simulink model "ProgrammingCalculator"  (R2021a)
settings: Solver=FixedStepDiscrete  StartTime=0.0  StopTime=10.0  RelTol=1e-3  EnableMultiTasking=on
libraries: simulink x6
settings Model: Creator=Karim  LastModifiedBy=Karim
settings DataIOCC: ReturnWorkspaceOutputs=off
settings OptimizationCC: DefaultParameterBehavior=Inlined  InlineInvariantSignals=on  EnableMemcpy=off  LifeSpan=1  EfficientTunableParamExpr=on
settings DebuggingCC: UnderspecifiedInitializationDetection=Classic  MergeDetectMultiDrivingBlocksExec=none  SFMachineParentedDataDiag=warning  ArithmeticOperatorsInVariantConditions=warning
settings ModelReferenceCC: PropagateSignalLabelsOutOfModel=off
settings SFSimCC: MATLABDynamicMemAlloc=off  CustomCodeUndefinedFunction=UseInterfaceOnly
settings RTWCC: SystemTargetFile=ert.tlc  GenCodeOnly=on  TemplateMakefile=ert_default_tmf  GenerateReport=on  IncludeHyperlinkInReport=on  LaunchReport=on  GenerateTraceInfo=on  GenerateTraceReport=on  GenerateTraceReportSl=on  GenerateTraceReportSf=on  GenerateTraceReportEml=on
settings CodeAppCC: ForceParamTrailComments=on  IgnoreCustomStorageClasses=off  OperatorAnnotations=on  SimulinkDataObjDesc=on  SFDataObjDesc=on  MATLABFcnDesc=on  InsertBlockDesc=on  StateflowObjectComments=on  MATLABSourceComments=on
settings ERTTargetCC: MultiwordLength=2048  GenerateSampleERTMain=on  InlinedParameterPlacement=NonHierarchical  ERTCustomFileTemplate=example_file_process.tlc

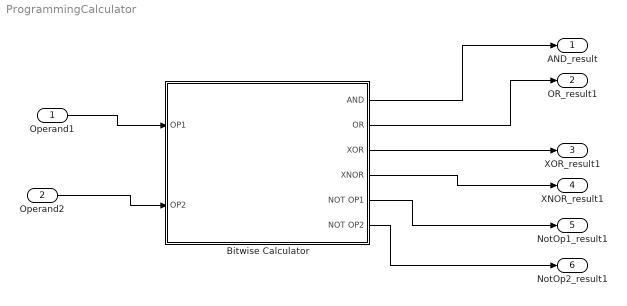
== system ProgrammingCalculator ==
  Operand1 : Inport
  Operand2 : Inport  Port=2
  Bitwise Calculator : Subsystem
  AND_result : Outport
  OR_result1 : Outport  Port=2
  XOR_result1 : Outport  Port=3
  XNOR_result1 : Outport  Port=4
  NotOp1_result1 : Outport  Port=5
  NotOp2_result1 : Outport  Port=6
  wires:
  Bitwise Calculator/1(AND) -> AND_result/1
  Bitwise Calculator/2(OR) -> OR_result1/1
  Bitwise Calculator/3(XOR) -> XOR_result1/1
  Bitwise Calculator/4(XNOR) -> XNOR_result1/1
  Bitwise Calculator/5(NOT OP1) -> NotOp1_result1/1
  Bitwise Calculator/6(NOT OP2) -> NotOp2_result1/1
  Operand1/1 -> Bitwise Calculator/1(OP1)
  Operand2/1 -> Bitwise Calculator/2(OP2)

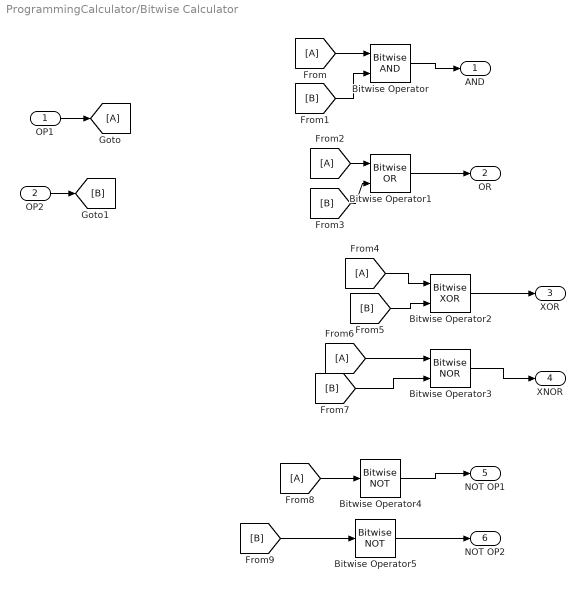
== system ProgrammingCalculator/Bitwise Calculator ==
  OP1 : Inport  OutDataTypeStr=uint16
  OP2 : Inport  Port=2  OutDataTypeStr=uint16
  Bitwise Operator : simulink/Logic and Bit Operations/Bitwise Operator  logicop=AND  UseBitMask=off  NumInputPorts=2  BitMask=bin2dec('11011001')  BitMaskRealWorld=Stored Integer
  Bitwise Operator1 : simulink/Logic and Bit Operations/Bitwise Operator  logicop=OR  UseBitMask=off  NumInputPorts=2  BitMask=bin2dec('11011001')  BitMaskRealWorld=Stored Integer
  Bitwise Operator2 : simulink/Logic and Bit Operations/Bitwise Operator  logicop=XOR  UseBitMask=off  NumInputPorts=2  BitMask=bin2dec('11011001')  BitMaskRealWorld=Stored Integer
  Bitwise Operator3 : simulink/Logic and Bit Operations/Bitwise Operator  logicop=NOR  UseBitMask=off  NumInputPorts=2  BitMask=bin2dec('11011001')  BitMaskRealWorld=Stored Integer
  Bitwise Operator4 : simulink/Logic and Bit Operations/Bitwise Operator  logicop=NOT  UseBitMask=off  BitMask=bin2dec('11011001')  BitMaskRealWorld=Stored Integer
  Bitwise Operator5 : simulink/Logic and Bit Operations/Bitwise Operator  logicop=NOT  UseBitMask=off  BitMask=bin2dec('11011001')  BitMaskRealWorld=Stored Integer
  AND : Outport
  OR : Outport  Port=2
  XOR : Outport  Port=3
  XNOR : Outport  Port=4
  NOT OP1 : Outport  Port=5
  NOT OP2 : Outport  Port=6
  wires:
  OP1/1 -> [A]
  Bitwise Operator/1 -> AND/1
  Bitwise Operator1/1 -> OR/1
  Bitwise Operator2/1 -> XOR/1
  Bitwise Operator3/1 -> XNOR/1
  OP2/1 -> [B]
  [A] -> Bitwise Operator/1
  [B] -> Bitwise Operator/2
  [A] -> Bitwise Operator1/1
  [B] -> Bitwise Operator1/2
  [A] -> Bitwise Operator2/1
  [B] -> Bitwise Operator2/2
  [A] -> Bitwise Operator3/1
  [B] -> Bitwise Operator3/2
  Bitwise Operator5/1 -> NOT OP2/1
  [B] -> Bitwise Operator5/1
  [A] -> Bitwise Operator4/1
  Bitwise Operator4/1 -> NOT OP1/1
